simulink model "DCmotor08"  (R2019b)
settings: Solver=ode45  StartTime=0.0  StopTime=0.5  MaxStep=1e-6  RelTol=1e-3
undefined symbols (not defined in the file): IaN, nN, TA, Tfn
libraries: powerlib x11, simulink x1
Description:
  | 转速闭环
settings Model: Creator=DELL  LastModifiedBy=Inspiron
settings DataIOCC: ReturnWorkspaceOutputs=off
settings DebuggingCC: ArithmeticOperatorsInVariantConditions=warning
settings SFSimCC: SimUseLocalCustomCode=off  CustomCodeUndefinedFunction=UseInterfaceOnly
settings RTWCC: RTWUseLocalCustomCode=off
settings CodeAppCC: StateflowObjectComments=on
settings SimscapeCC: SimscapeNormalizeSystem=off

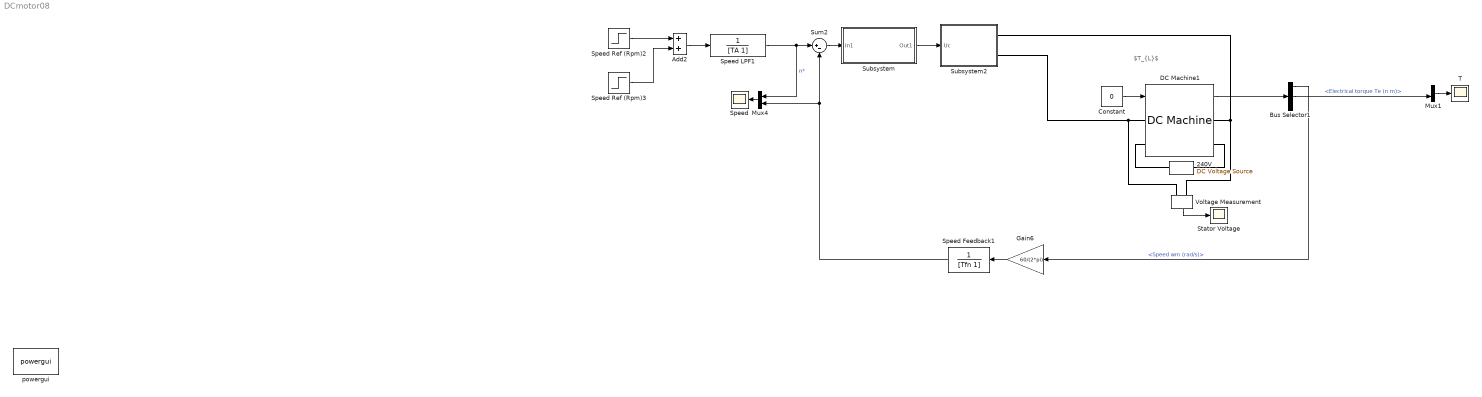
== system DCmotor08 ==
  note: $T_{L}$
  240V : powerlib/Electrical Sources/DC Voltage Source  Amplitude=240  Measurements=None
      settings: SourceProductName=Simscape Electrical
  Add2 : Sum
  Bus Selector1 : BusSelector  OutputSignals=Speed wm (rad/s),Electrical torque Te (n m),Armature current ia (A)
  Constant : Constant  Value=0
  DC Machine1 : powerlib/Machines/DC Machine  PresetModel=No  MechanicalLoad=Torque TL  FieldType=Wound  ShowDetailedParameters=on  MeasurementBus=off  RLa="[ 0.6  0.012]"  RLf="[ 240  120]"  Laf=1.8  MachineConstant=Torque constant (N.m/A)  Ke=1.8  Kt=1.8  J=0.05  Bm=0  Tf=0  w0=1  Ifinit=1  TsPowergui=0  TsBlock=-1
      settings: SourceProductName=Simscape Electrical
  Gain6 : Gain  Gain=60/(2*pi)
  Mux1 : Mux  Inputs=2
  Mux4 : Mux  Inputs=2
  Speed : Scope
  Speed Feedback1 : TransferFcn  Denominator=[Tfn 1]
  Speed LPF1 : TransferFcn  Denominator=[TA 1]
  Speed Ref (Rpm)2 : Step  Time=0.05  After=0.8*nN  SampleTime=0
  Speed Ref (Rpm)3 : Step  Time=0.4  After=-0.3*nN  SampleTime=0  VectorParams1D=off
  Stator Voltage : Scope
  Subsystem : Subsystem
  Subsystem2 : Subsystem
  Sum2 : Sum  Inputs=|+-
  T : Scope
  Voltage Measurement : powerlib/Measurements/Voltage Measurement  PhasorSimulation=off  OutputType=Complex  PSBequivalent=0
      settings: SourceProductName=Simscape Electrical
  powergui : powerlib/powergui  Priority=1  SimulationMode=Continuous  SampleTime=50e-6  frequency=60  Iterations=50  frequencyindice=0  Pbase=100e6  ErrMax=1e-4  UnitsV=kV  UnitsW=MW  buscounter=0  FunctionMessages=off  echomessages=off  EnableUseOfTLC=off  CurrentSourceSwitches=on  DisableSnubberDevices=off  DisableRonSwitches=off  DisableVfSwitches=off  DisplayEquations=off  AutomaticDiscreteSolvers=off  SolverType=Tustin/Backward Euler (TBE)  Interpol=off  ExternalGateDelay=off  methode=off  Ts=10  x0status=blocks  SPID=off  SwTol=0  HookPort=off  NonlinearTolerance=1e-4  nMaxIteration=100  ContinueOnMaxIteration=off  RestoreLinks=warning  ResistiveCurrentMeasurement=off  Frange=[0:2:500]  Ylog=off  Xlog=on  ShowGrid=off  save=off  variable=ZData  structure=0  ZoomFFT=off  StartTime=0.0  cycles=1  DisplayStyle=1  fundamental=60  FreqAxis=off  MaxFrequency=1000  frequencyindicesteady=1  RmsSteady=1  display=off
      settings: SourceProductName=Simscape Electrical
  wires:
  Speed Ref (Rpm)2/1 -> Add2/1
  Speed Ref (Rpm)3/1 -> Add2/2
  Sum2/1 -> Subsystem/1(In1)
  DC Machine1/1 -> Bus Selector1/1
  Add2/1 -> Speed LPF1/1
  Gain6/1 -> Speed Feedback1/1
  Voltage Measurement/1 -> Stator Voltage/1
  Bus Selector1/1 -> Gain6/1  "<Speed wm (rad/s)>"
  Speed Feedback1/1 -> Sum2/2, Mux4/2
  Mux4/1 -> Speed/1
  Speed LPF1/1 -> Sum2/1, Mux4/1  "n*"
  Constant/1 -> DC Machine1/1
  Bus Selector1/2 -> Mux1/2  "<Electrical torque Te (n m)>"
  ? -> Mux1/1  "TL"
  Mux1/1 -> T/1
  Subsystem/1(Out1) -> Subsystem2/1(Uc)
  connections:
  240V/RConn1 -- DC Machine1/LConn2
  240V/LConn1 -- DC Machine1/RConn2
  DC Machine1/LConn1 -- Voltage Measurement/LConn1 -- Subsystem2/RConn2
  DC Machine1/RConn1 -- Voltage Measurement/LConn2 -- Subsystem2/RConn1

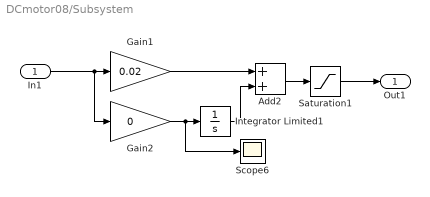
== system DCmotor08/Subsystem ==
  In1 : Inport
  Add2 : Sum
  Gain1 : Gain  Gain=0.02
  Gain2 : Gain  Gain=0
  Integrator Limited1 : Integrator  LimitOutput=on  UpperSaturationLimit=2*IaN  LowerSaturationLimit=0
  Saturation1 : Saturate  UpperLimit=2*IaN  LowerLimit=-2*IaN
  Scope6 : Scope
  Out1 : Outport
  wires:
  Gain1/1 -> Add2/1
  In1/1 -> Gain1/1, Gain2/1
  Saturation1/1 -> Out1/1
  Gain2/1 -> Scope6/1, Integrator Limited1/1
  Integrator Limited1/1 -> Add2/2
  Add2/1 -> Saturation1/1

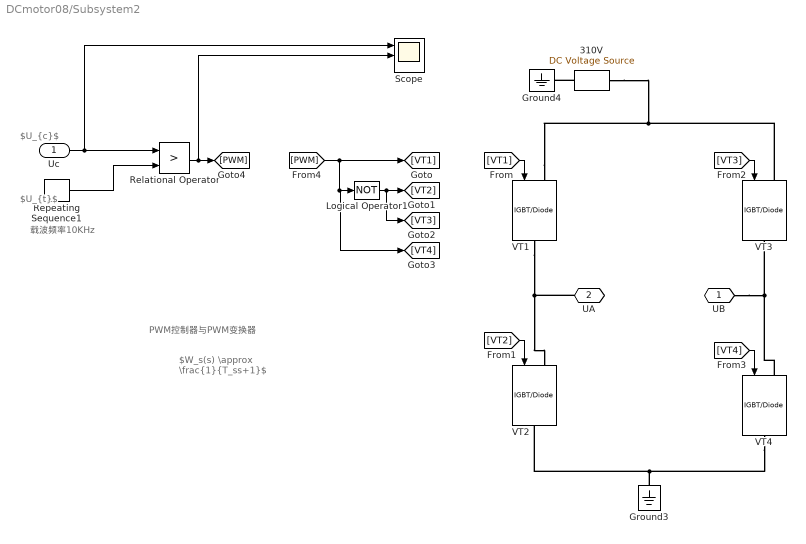
== system DCmotor08/Subsystem2 ==
  note: 载波频率10KHz
  note: $U_{c}$
  note: $U_{t}$
  note: $W_s(s) \approx \frac{1}{T_ss+1}$
  note: PWM控制器与PWM变换器
  Uc : Inport
  310V : powerlib/Electrical Sources/DC Voltage Source  Amplitude=310  Measurements=None
      settings: SourceProductName=Simscape Electrical
  Ground3 : powerlib/Elements/Ground  LConnTagsString=a
      settings: SourceProductName=Simscape Electrical
  Ground4 : powerlib/Elements/Ground  LConnTagsString=a
      settings: SourceProductName=Simscape Electrical
  Logical Operator1 : Logic  Operator=NOT  AllPortsSameDT=off  OutDataTypeStr=boolean
  Relational Operator : RelationalOperator  Operator=>  OutDataTypeStr=boolean  RndMeth=Simplest
  Repeating Sequence1 : simulink/Sources/Repeating Sequence  rep_seq_t=[0 1e-4 ]  rep_seq_y=[-5 5]
  Scope : Scope  NumInputPorts=3
  VT{1..4} (4 alike) : powerlib/Power Electronics/IGBT//Diode  Ron=1e-3  Rs=1e5  Cs=inf  Measurements=off
      settings: SourceProductName=Simscape Electrical
  UB : PMIOPort  Side=Right
  UA : PMIOPort  Port=2  Side=Right
  wires:
  Logical Operator1/1 -> [VT3], [VT2]
  [PWM] -> [VT4], Logical Operator1/1, [VT1]
  [VT2] -> VT2/1
  [VT4] -> VT4/1
  [VT3] -> VT3/1
  [VT1] -> VT1/1
  Repeating Sequence1/1 -> Relational Operator/2
  Uc/1 -> Scope/1, Relational Operator/1
  Relational Operator/1 -> Scope/2, [PWM]
  connections:
  VT1/RConn1 -- VT2/LConn1 -- UA/RConn1
  310V/LConn1 -- Ground4/LConn1
  VT4/LConn1 -- UB/RConn1 -- VT3/RConn1
  VT1/LConn1 -- VT3/LConn1 -- 310V/RConn1
  VT2/RConn1 -- VT4/RConn1 -- Ground3/LConn1
